simulink model "RsCalculation"  (R2025b)
settings: Solver=FixedStepDiscrete  StartTime=0.0  StopTime=10.0  RelTol=1e-3
model workspace (MAT data in the model file):
  R_base = Simulink.Parameter
  R_base.Value = 0.02
  R_base.Complexity = 'real'
  R_base.Dimensions = [1 1]
  R_base.DataType = 'auto'
  T_Coeff = Simulink.Parameter
  T_Coeff.Value = 0.00393
  T_Coeff.Complexity = 'real'
  T_Coeff.Dimensions = [1 1]
  T_Coeff.DataType = 'auto'
  T_base = Simulink.Parameter
  T_base.Value = 25
  T_base.Complexity = 'real'
  T_base.Dimensions = [1 1]
  T_base.DataType = 'auto'
settings Model: DataDictionary=TractionEmotorSoftwareArchInterfaceData.sldd  Creator=dakaihu  LastModifiedBy=dakaihu
settings OptimizationCC: DefaultParameterBehavior=Inlined  GainParamInheritBuiltInType=on  UseFloatMulNetSlope=on  InlineInvariantSignals=on  PassReuseOutputArgsAs=Individual arguments  ZeroExternalMemoryAtStartup=off  ZeroInternalMemoryAtStartup=off  NoFixptDivByZeroProtection=on  EfficientFloat2IntCast=on  LifeSpan=1  OptimizeBlockOrder=speed  DifferentSizesBufferReuse=on  EfficientTunableParamExpr=on
settings DebuggingCC: SignalInfNanChecking=warning  CheckMatrixSingularityMsg=error  IntegerOverflowMsg=error  ParameterTunabilityLossMsg=error  UnconnectedInputMsg=warning  UnconnectedOutputMsg=warning  UnconnectedLineMsg=warning  UniqueDataStoreMsg=warning  IntegerSaturationMsg=error
settings HardwareCC: ProdBitPerChar=16.0  ProdBitPerInt=16.0  ProdBitPerPointer=32.0  ProdBitPerSizeT=32.0  ProdBitPerPtrDiffT=32.0  ProdLargestAtomicInteger=Integer  ProdLargestAtomicFloat=None  ProdWordSize=16.0  ProdLongLongMode=on  ProdHWDeviceType=Texas Instruments->C2000
settings SFSimCC: MATLABDynamicMemAlloc=off
settings RTWCC: SystemTargetFile=ert.tlc  GenCodeOnly=on  TemplateMakefile=ert_default_tmf  Description=Embedded Coder
settings CodeAppCC: ForceParamTrailComments=on  IgnoreCustomStorageClasses=off  OperatorAnnotations=on  SimulinkDataObjDesc=on  SFDataObjDesc=on  CustomSymbolStrGlobalVar=rt$N$M  CustomSymbolStrType=$N$M  CustomSymbolStrFcn=$N$M$F  CustomSymbolStrMacro=$N$M  InsertBlockDesc=on
settings ERTTargetCC: ERTCustomFileTemplate=example_file_process.tlc  ERTFilePackagingFormat=CompactWithDataFile  TargetLangStandard=C99 (ISO)  GenerateSampleERTMain=on  IncludeMdlTerminateFcn=off  CombineSignalStateStructs=on  SuppressErrorStatus=on  SupportAbsoluteTime=off  SupportComplex=off

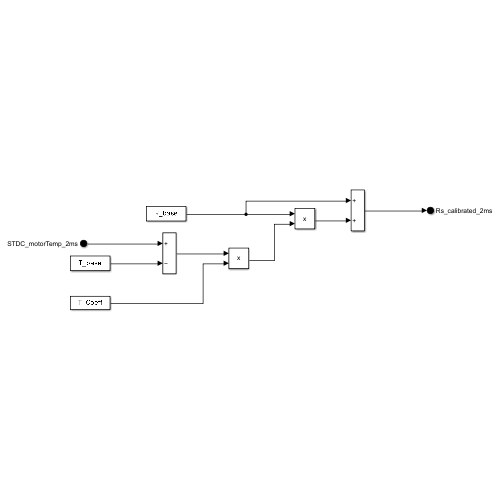
[thumbnail: Simulink's stored preview of the top-level diagram]
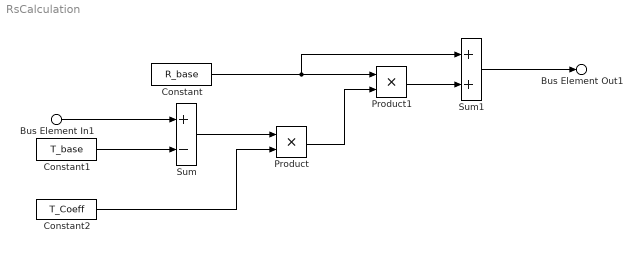
== system RsCalculation ==
  Bus Element In1 : Inport  PortName=STDC_motorTemp_2ms
  Constant : Constant  Value=R_base
  Constant1 : Constant  Value=T_base  SampleTime=-1
  Constant2 : Constant  Value=T_Coeff  SampleTime=-1
  Product : Product
  Product1 : Product
  Sum : Sum  Inputs=+-
  Sum1 : Sum
  Bus Element Out1 : Outport  PortName=Rs_calibrated_2ms
  wires:
  Constant1/1 -> Sum/2
  Bus Element In1/1 -> Sum/1
  Sum/1 -> Product/1
  Constant2/1 -> Product/2
  Product/1 -> Product1/2
  Constant/1 -> Sum1/1, Product1/1
  Product1/1 -> Sum1/2
  Sum1/1 -> Bus Element Out1/1
